simulink subsystem "Plant"  (R2023b)
settings: Solver=VariableStepAuto  StartTime=0.0  StopTime=10.0  RelTol=1e-3
undefined symbols (not defined in the file): BPlantSoCReset, DiscIntNeverNeededParam, rCellCapacity, rInitialSoC, tSim
settings Model: DataDictionary=ElectricPowertrain_data.sldd  EnableAccessToBaseWorkspace=off  Creator=Elio  LastModifiedBy=Elio

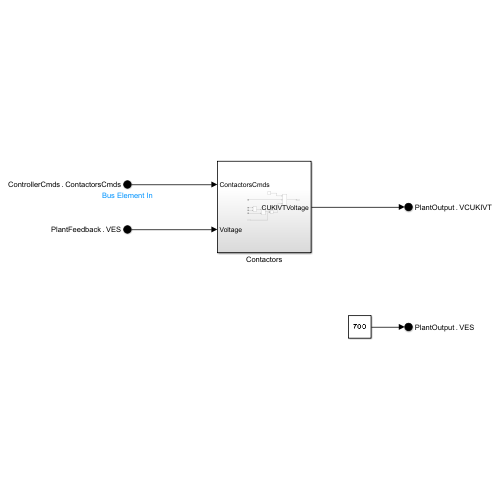
[thumbnail: Simulink's stored preview of the top-level diagram]
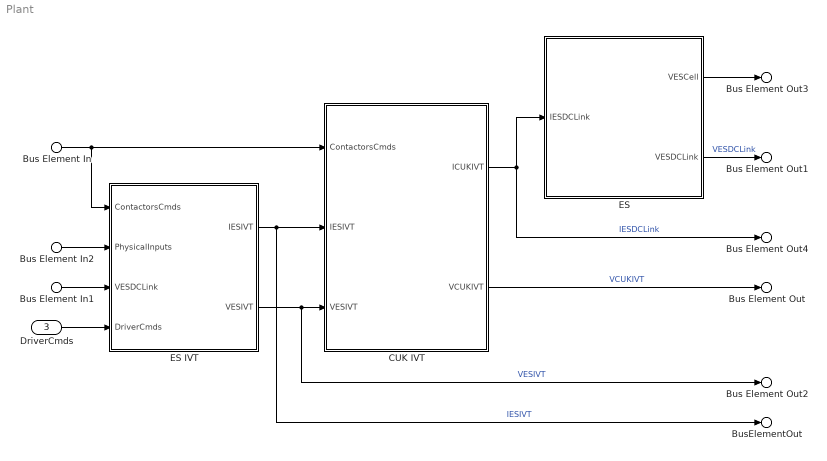
== system Plant ==
  Bus Element In2 : Inport  PortName=PhysicalInputs
  Bus Element In : Inport  Port=2  PortName=ControllerCmds  Element=ContactorsCmds
  DriverCmds : Inport  Port=3
  Bus Element In1 : Inport  Port=4  PortName=PlantFeedback  Element=VESDCLink
  CUK IVT : Subsystem
  ES : Subsystem
  ES IVT : Subsystem
  Bus Element Out : Outport  PortName=PlantOutput  Element=VCUKIVT
  BusElementOut : Outport  PortName=PlantOutput  Element=IESIVT
  Bus Element Out1 : Outport  PortName=PlantOutput  Element=VESDCLink
  Bus Element Out2 : Outport  PortName=PlantOutput  Element=VESIVT
  Bus Element Out3 : Outport  PortName=PlantOutput  Element=VESCell
  Bus Element Out4 : Outport  PortName=PlantOutput  Element=ICUKIVT
  wires:
  Bus Element In/1 -> CUK IVT/1(ContactorsCmds), ES IVT/1(ContactorsCmds)
  CUK IVT/2(VCUKIVT) -> Bus Element Out/1  "VCUKIVT"
  Bus Element In1/1 -> ES IVT/3(VESDCLink)
  ES IVT/2(VESIVT) -> Bus Element Out2/1, CUK IVT/3(VESIVT)  "VESIVT"
  Bus Element In2/1 -> ES IVT/2(PhysicalInputs)
  ES/2(VESDCLink) -> Bus Element Out1/1  "VESDCLink"
  ES/1(VESCell) -> Bus Element Out3/1
  CUK IVT/1(ICUKIVT) -> Bus Element Out4/1, ES/1(IESDCLink)  "IESDCLink"
  DriverCmds/1 -> ES IVT/4(DriverCmds)
  ES IVT/1(IESIVT) -> CUK IVT/2(IESIVT), BusElementOut/1  "IESIVT"

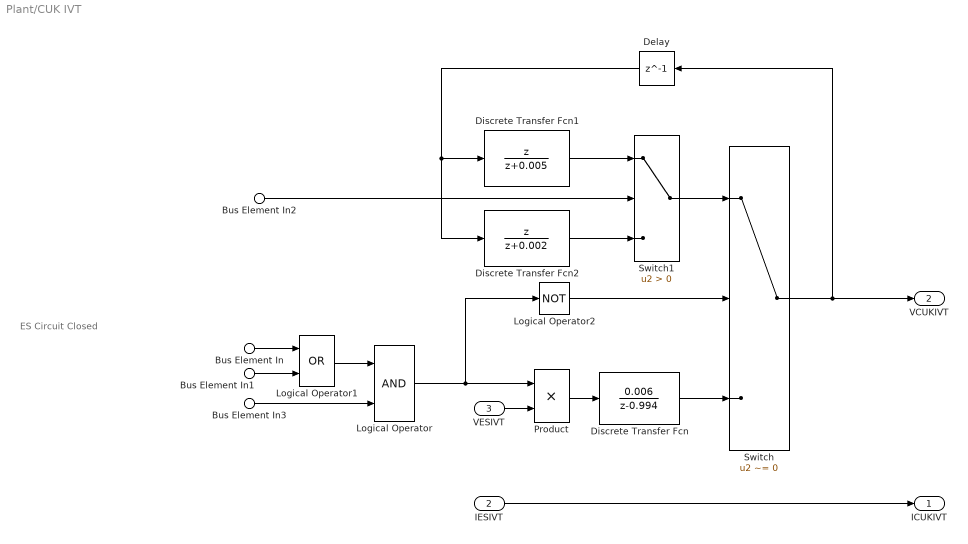
== system Plant/CUK IVT ==
  note: ES Circuit Closed
  Bus Element In : Inport  PortName=ContactorsCmds  Element=BContPosRequested
  Bus Element In3 : Inport  PortName=ContactorsCmds  Element=BContNegRequested
  Bus Element In1 : Inport  PortName=ContactorsCmds  Element=BPrechargeRequested
  Bus Element In2 : Inport  PortName=ContactorsCmds  Element=BActiveDischargeRequested
  IESIVT : Inport  Port=2
  VESIVT : Inport  Port=3
  Delay : Delay  DelayLength=1
  Discrete Transfer Fcn : DiscreteTransferFcn  Numerator=[0.006]  Denominator=[1 -0.994]
  Discrete Transfer Fcn1 : DiscreteTransferFcn  Numerator=[1 0]  Denominator=[1 0.005]
  Discrete Transfer Fcn2 : DiscreteTransferFcn  Numerator=[1 0]  Denominator=[1 0.002]
  Logical Operator : Logic  AllPortsSameDT=off  OutDataTypeStr=boolean
  Logical Operator1 : Logic  Operator=OR  AllPortsSameDT=off  OutDataTypeStr=boolean
  Logical Operator2 : Logic  Operator=NOT  AllPortsSameDT=off  OutDataTypeStr=boolean
  Product : Product
  Switch : Switch  Criteria=u2 ~= 0  SaturateOnIntegerOverflow=off  InputSameDT=off
  Switch1 : Switch  Criteria=u2 > Threshold  SaturateOnIntegerOverflow=off  InputSameDT=off
  ICUKIVT : Outport
  VCUKIVT : Outport  Port=2
  wires:
  IESIVT/1 -> ICUKIVT/1
  Logical Operator2/1 -> Switch/2
  Discrete Transfer Fcn2/1 -> Switch1/3
  Discrete Transfer Fcn1/1 -> Switch1/1
  Switch1/1 -> Switch/1
  Logical Operator/1 -> Logical Operator2/1, Product/1
  Bus Element In2/1 -> Switch1/2
  Delay/1 -> Discrete Transfer Fcn2/1, Discrete Transfer Fcn1/1
  Discrete Transfer Fcn/1 -> Switch/3
  Bus Element In/1 -> Logical Operator1/1
  Bus Element In1/1 -> Logical Operator1/2
  Logical Operator1/1 -> Logical Operator/1
  Bus Element In3/1 -> Logical Operator/2
  VESIVT/1 -> Product/2
  Product/1 -> Discrete Transfer Fcn/1
  Switch/1 -> Delay/1, VCUKIVT/1

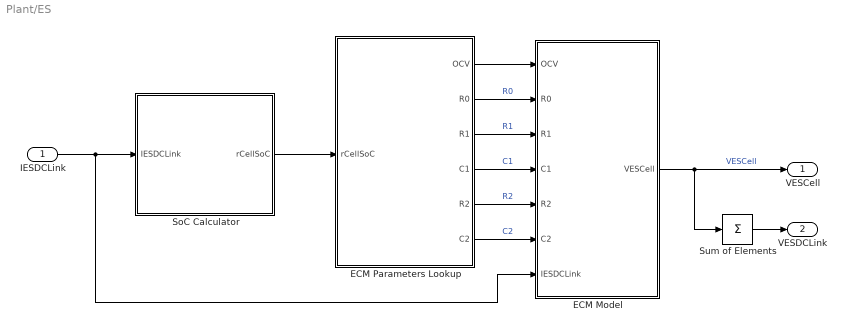
== system Plant/ES ==
  IESDCLink : Inport
  ECM Model : Subsystem
  ECM Parameters Lookup : Subsystem
  SoC Calculator : Subsystem
  Sum of Elements : Sum  Inputs=+
  VESCell : Outport
  VESDCLink : Outport  Port=2
  wires:
  IESDCLink/1 -> ECM Model/7(IESDCLink), SoC Calculator/1(IESDCLink)
  Sum of Elements/1 -> VESDCLink/1
  ECM Model/1(VESCell) -> VESCell/1, Sum of Elements/1  "VESCell"
  ECM Parameters Lookup/6(C2) -> ECM Model/6(C2)  "C2"
  ECM Parameters Lookup/5(R2) -> ECM Model/5(R2)  "R2"
  ECM Parameters Lookup/4(C1) -> ECM Model/4(C1)  "C1"
  ECM Parameters Lookup/3(R1) -> ECM Model/3(R1)  "R1"
  ECM Parameters Lookup/2(R0) -> ECM Model/2(R0)  "R0"
  ECM Parameters Lookup/1(OCV) -> ECM Model/1(OCV)
  SoC Calculator/1(rCellSoC) -> ECM Parameters Lookup/1(rCellSoC)

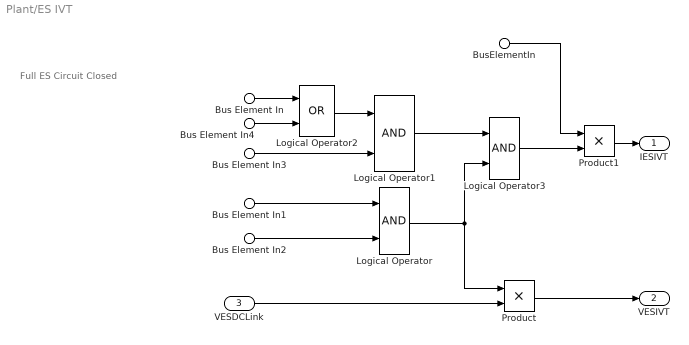
== system Plant/ES IVT ==
  note: Full ES Circuit Closed
  Bus Element In : Inport  PortName=ContactorsCmds  Element=BContPosRequested
  Bus Element In3 : Inport  PortName=ContactorsCmds  Element=BContNegRequested
  Bus Element In4 : Inport  PortName=ContactorsCmds  Element=BPrechargeRequested
  Bus Element In1 : Inport  Port=2  PortName=PhysicalInputs  Element=BServiceDisconnectPos
  Bus Element In2 : Inport  Port=2  PortName=PhysicalInputs  Element=BServiceDisconnectNeg
  VESDCLink : Inport  Port=3
  BusElementIn : Inport  Port=4  PortName=DriverCmds  Element=IESDCLink
  Logical Operator : Logic  AllPortsSameDT=off  OutDataTypeStr=boolean
  Logical Operator1 : Logic  AllPortsSameDT=off  OutDataTypeStr=boolean
  Logical Operator2 : Logic  Operator=OR  AllPortsSameDT=off  OutDataTypeStr=boolean
  Logical Operator3 : Logic  AllPortsSameDT=off  OutDataTypeStr=boolean
  Product : Product
  Product1 : Product
  IESIVT : Outport
  VESIVT : Outport  Port=2
  wires:
  Product1/1 -> IESIVT/1
  BusElementIn/1 -> Product1/1
  Logical Operator3/1 -> Product1/2
  Logical Operator1/1 -> Logical Operator3/1
  Bus Element In3/1 -> Logical Operator1/2
  Bus Element In4/1 -> Logical Operator2/2
  Bus Element In/1 -> Logical Operator2/1
  Logical Operator2/1 -> Logical Operator1/1
  Product/1 -> VESIVT/1
  Logical Operator/1 -> Logical Operator3/2, Product/1
  Bus Element In2/1 -> Logical Operator/2
  Bus Element In1/1 -> Logical Operator/1
  VESDCLink/1 -> Product/2

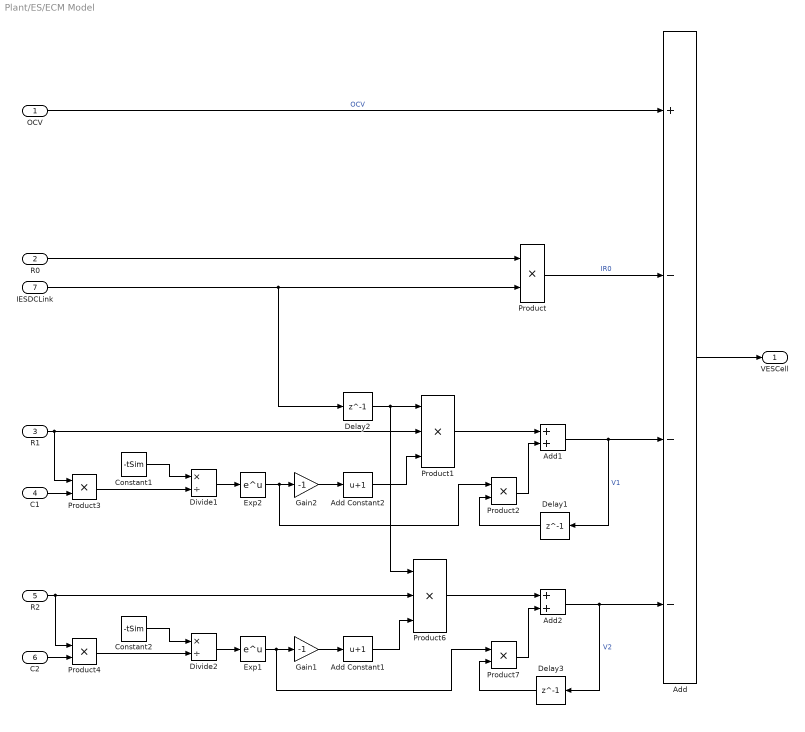
== system Plant/ES/ECM Model ==
  OCV : Inport
  R0 : Inport  Port=2
  R1 : Inport  Port=3
  C1 : Inport  Port=4
  R2 : Inport  Port=5
  C2 : Inport  Port=6
  IESDCLink : Inport  Port=7
  Add : Sum  Inputs=+---
  Add Constant1 : Bias  Bias=1  SaturateOnIntegerOverflow=off
  Add Constant2 : Bias  Bias=1  SaturateOnIntegerOverflow=off
  Add1 : Sum
  Add2 : Sum
  Constant1 : Constant  Value=-tSim  SampleTime=tSim
  Constant2 : Constant  Value=-tSim  SampleTime=tSim
  Delay1 : Delay  DelayLength=1
  Delay2 : Delay  DelayLength=1
  Delay3 : Delay  DelayLength=1
  Divide1 : Product  Inputs=*/
  Divide2 : Product  Inputs=*/
  Exp1 : Math
  Exp2 : Math
  Gain1 : Gain  Gain=-1
  Gain2 : Gain  Gain=-1
  Product{,2..4,7} (5 alike) : Product
  Product1 : Product  Inputs=3
  Product6 : Product  Inputs=3
  VESCell : Outport
  wires:
  Delay2/1 -> Product6/1, Product1/1
  R2/1 -> Product6/2, Product4/1
  C2/1 -> Product4/2
  Product4/1 -> Divide2/2
  Product3/1 -> Divide1/2
  C1/1 -> Product3/2
  Gain2/1 -> Add Constant2/1
  Add Constant2/1 -> Product1/3
  R1/1 -> Product1/2, Product3/1
  Divide1/1 -> Exp2/1
  Add1/1 -> Delay1/1, Add/3  "V1"
  Constant1/1 -> Divide1/1
  Exp2/1 -> Gain2/1, Product2/1
  Product2/1 -> Add1/2
  Delay1/1 -> Product2/2
  Product1/1 -> Add1/1
  Product7/1 -> Add2/2
  Add Constant1/1 -> Product6/3
  IESDCLink/1 -> Delay2/1, Product/2
  Product6/1 -> Add2/1
  Add2/1 -> Add/4, Delay3/1  "V2"
  Exp1/1 -> Gain1/1, Product7/1
  Constant2/1 -> Divide2/1
  Divide2/1 -> Exp1/1
  Gain1/1 -> Add Constant1/1
  Delay3/1 -> Product7/2
  Add/1 -> VESCell/1
  Product/1 -> Add/2  "IR0"
  OCV/1 -> Add/1  "OCV"
  R0/1 -> Product/1

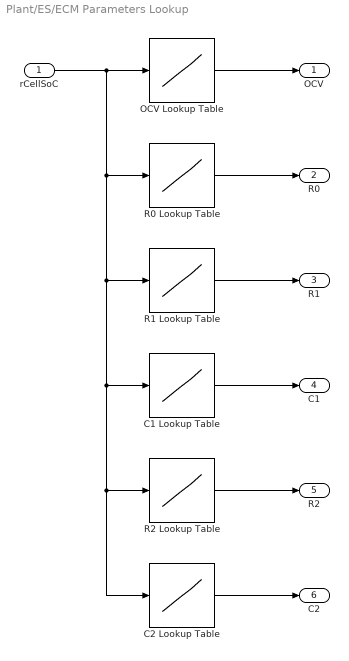
== system Plant/ES/ECM Parameters Lookup ==
  rCellSoC : Inport
  C1 Lookup Table : Lookup_n-D  NumberOfTableDimensions=1  LookupTableObject=''  BreakpointsForDimension1=[0 10 20 30 40 50 60 70 80 90 100]  BreakpointsForDimension1FirstPoint=10  BreakpointsForDimension2FirstPoint=10  BreakpointsForDimension1Spacing=12  BreakpointsForDimension2Spacing=12  IndexSearchMethod=Evenly spaced points  Table=[1295651.21966291;1295651.21966291;1753730.04539165;2232989.02220951;1322336.33589948;1761750.56589617;1404185.19646928;1377060.54214332;946091.464996784;2605207.70539984;2605207.70539984]  DiagnosticForOutOfRangeInput=Error  InternalRulePriority=Speed  RndMeth=Simplest
  C2 Lookup Table : Lookup_n-D  NumberOfTableDimensions=1  LookupTableObject=''  BreakpointsForDimension1=[0 10 20 30 40 50 60 70 80 90 100]  BreakpointsForDimension1FirstPoint=10  BreakpointsForDimension2FirstPoint=10  BreakpointsForDimension1Spacing=12  BreakpointsForDimension2Spacing=12  IndexSearchMethod=Evenly spaced points  Table=[25640.9009821787;25640.9009821787;32135.7617897906;32135.7617897906;37289.3370479989;34003.1851136664;26539.6688237942;31883.6430599253;28172.9896038947;23205.4641188252;23205.4641188252]  DiagnosticForOutOfRangeInput=Error  InternalRulePriority=Speed  RndMeth=Simplest
  OCV Lookup Table : Lookup_n-D  NumberOfTableDimensions=1  LookupTableObject=''  BreakpointsForDimension1=[0, 10, 20, 30, 40, 50, 60, 70, 80, 90, 100]  BreakpointsForDimension1FirstPoint=10  BreakpointsForDimension2FirstPoint=10  BreakpointsForDimension1Spacing=12  BreakpointsForDimension2Spacing=12  Table=[2.8; 3.531; 3.723; 3.802; 3.869; 3.909; 3.949; 3.984; 4.048; 4.086; 4.182]  DiagnosticForOutOfRangeInput=Error  InternalRulePriority=Speed  RndMeth=Simplest
  R0 Lookup Table : Lookup_n-D  NumberOfTableDimensions=1  LookupTableObject=''  BreakpointsForDimension1=[0;10;20;30;40;50;60;70;80;90;100]  BreakpointsForDimension1FirstPoint=10  BreakpointsForDimension2FirstPoint=10  BreakpointsForDimension1Spacing=12  BreakpointsForDimension2Spacing=12  IndexSearchMethod=Evenly spaced points  Table=[0.00163076923076923;0.00163076923076923;0.0016;0.0016;0.0016;0.00156923076923077;0.00156923076923076;0.00163076923076923;0.00160000000000002;0.00179869881362418;0.00179869881362418]  DiagnosticForOutOfRangeInput=Error  InternalRulePriority=Speed  RndMeth=Simplest
  R1 Lookup Table : Lookup_n-D  NumberOfTableDimensions=1  LookupTableObject=''  BreakpointsForDimension1=[0 10 20 30 40 50 60 70 80 90 100]  BreakpointsForDimension1FirstPoint=10  BreakpointsForDimension2FirstPoint=10  BreakpointsForDimension1Spacing=12  BreakpointsForDimension2Spacing=12  IndexSearchMethod=Evenly spaced points  Table=[0.00104727002001105;0.00104727002001105;0.000248441004746327;0.000218443681758313;0.000486442901157713;0.000400083406941612;0.000408297350218177;0.000354918952509598;0.000446729201021446;0.000283154825970381;0.000283154825970381]  DiagnosticForOutOfRangeInput=Error  InternalRulePriority=Speed  RndMeth=Simplest
  R2 Lookup Table : Lookup_n-D  NumberOfTableDimensions=1  LookupTableObject=''  BreakpointsForDimension1=[0 10 20 30 40 50 60 70 80 90 100]  BreakpointsForDimension1FirstPoint=10  BreakpointsForDimension2FirstPoint=10  BreakpointsForDimension1Spacing=12  BreakpointsForDimension2Spacing=12  IndexSearchMethod=Evenly spaced points  Table=[0.00102234226974734;0.00102234226974734;0.000911136914667474;0.000913748876974288;0.000953901562345974;0.000977217447154348;0.000853598634584605;0.00086117326499532;0.00110872164638919;0.00117402665432263;0.00117402665432263]  DiagnosticForOutOfRangeInput=Error  InternalRulePriority=Speed  RndMeth=Simplest
  OCV : Outport
  R0 : Outport  Port=2
  R1 : Outport  Port=3
  C1 : Outport  Port=4
  R2 : Outport  Port=5
  C2 : Outport  Port=6
  wires:
  C2 Lookup Table/1 -> C2/1
  R2 Lookup Table/1 -> R2/1
  C1 Lookup Table/1 -> C1/1
  R1 Lookup Table/1 -> R1/1
  R0 Lookup Table/1 -> R0/1
  OCV Lookup Table/1 -> OCV/1
  rCellSoC/1 -> OCV Lookup Table/1, R0 Lookup Table/1, C1 Lookup Table/1, R2 Lookup Table/1, C2 Lookup Table/1, R1 Lookup Table/1

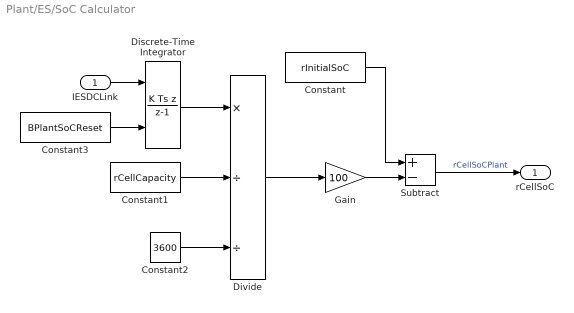
== system Plant/ES/SoC Calculator ==
  IESDCLink : Inport
  Constant : Constant  Value=rInitialSoC  SampleTime=tSim
  Constant1 : Constant  Value=rCellCapacity  SampleTime=tSim
  Constant2 : Constant  Value=3600  SampleTime=tSim
  Constant3 : Constant  Value=BPlantSoCReset  SampleTime=tSim
  Discrete-Time Integrator : DiscreteIntegrator  IntegratorMethod=Integration: Backward Euler  ExternalReset=rising  SampleTime=-1  ICPrevOutput=DiscIntNeverNeededParam  ICPrevScaledInput=DiscIntNeverNeededParam
  Divide : Product  Inputs=*//
  Gain : Gain  Gain=100
  Subtract : Sum  Inputs=+-
  rCellSoC : Outport
  wires:
  Constant3/1 -> Discrete-Time Integrator/2
  Constant2/1 -> Divide/3
  Subtract/1 -> rCellSoC/1  "rCellSoCPlant"
  Gain/1 -> Subtract/2
  Divide/1 -> Gain/1
  Constant1/1 -> Divide/2
  Discrete-Time Integrator/1 -> Divide/1
  Constant/1 -> Subtract/1
  IESDCLink/1 -> Discrete-Time Integrator/1
